simulink model "sim_6dof"  (R2025b)
settings: Solver=FixedStepAuto  StartTime=0.0  StopTime=30  FixedStep=0.005  RelTol=1e-3
InitFcn:
  | params_3dof
libraries: simulink_extras x1, simulink x1
settings Model: Creator=schwmaxi  LastModifiedBy=schwmaxi
settings OptimizationCC: UseDivisionForNetSlopeComputation=on  GainParamInheritBuiltInType=on  UseFloatMulNetSlope=on  EnhancedBackFolding=on  BooleansAsBitfields=on  PassReuseOutputArgsAs=Individual arguments  StateBitsets=on  DataBitsets=on  ZeroExternalMemoryAtStartup=off  ZeroInternalMemoryAtStartup=off  NoFixptDivByZeroProtection=on  EfficientFloat2IntCast=on  LifeSpan=1  OptimizeBlockOrder=speed  DifferentSizesBufferReuse=on  EfficientTunableParamExpr=on
settings DebuggingCC: ParameterTunabilityLossMsg=error
settings HardwareCC: ProdBitPerPointer=32.0  ProdBitPerSizeT=32.0  ProdBitPerPtrDiffT=32.0  ProdLargestAtomicFloat=None  ProdWordSize=32.0  ProdLongLongMode=on  ProdHWDeviceType=Custom Processor->Custom Processor
settings SFSimCC: MATLABDynamicMemAlloc=off  SimTargetLang=C++  SimDLTargetLibrary=mkl-dnn
settings RTWCC: SystemTargetFile=ert.tlc  GenCodeOnly=on  TemplateMakefile=ert_default_tmf  TargetLang=C++  Description=Embedded Coder
settings CodeAppCC: ForceParamTrailComments=on  IgnoreCustomStorageClasses=off  OperatorAnnotations=on  SimulinkDataObjDesc=on  SFDataObjDesc=on  CustomSymbolStrGlobalVar=rt$N$M  CustomSymbolStrType=$N$M  CustomSymbolStrFcn=$N$M$F  CustomSymbolStrMacro=$N$M  InsertBlockDesc=on
settings ERTTargetCC: InlinedParameterPlacement=Hierarchical  RootIOFormat=Structure reference  ERTCustomFileTemplate=example_file_process.tlc  ERTFilePackagingFormat=CompactWithDataFile  TargetLangStandard=C++11 (ISO)  GenerateSampleERTMain=on  IncludeMdlTerminateFcn=off  CombineSignalStateStructs=on  SupportAbsoluteTime=off  CodeInterfacePackaging=C++ class  SubcomponentCodeInterfacePackaging=C++ class  SupportComplex=off  SupportNonInlinedSFcns=on

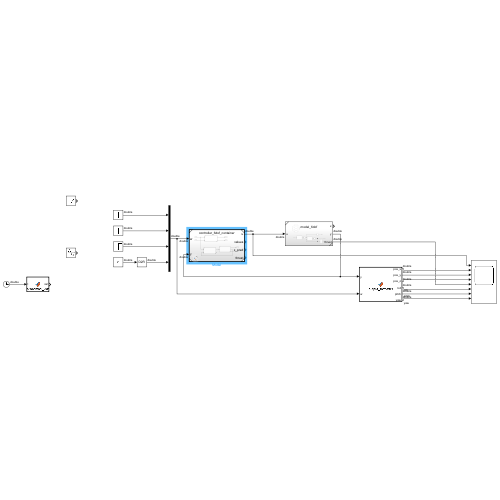
[thumbnail: Simulink's stored preview of the top-level diagram]
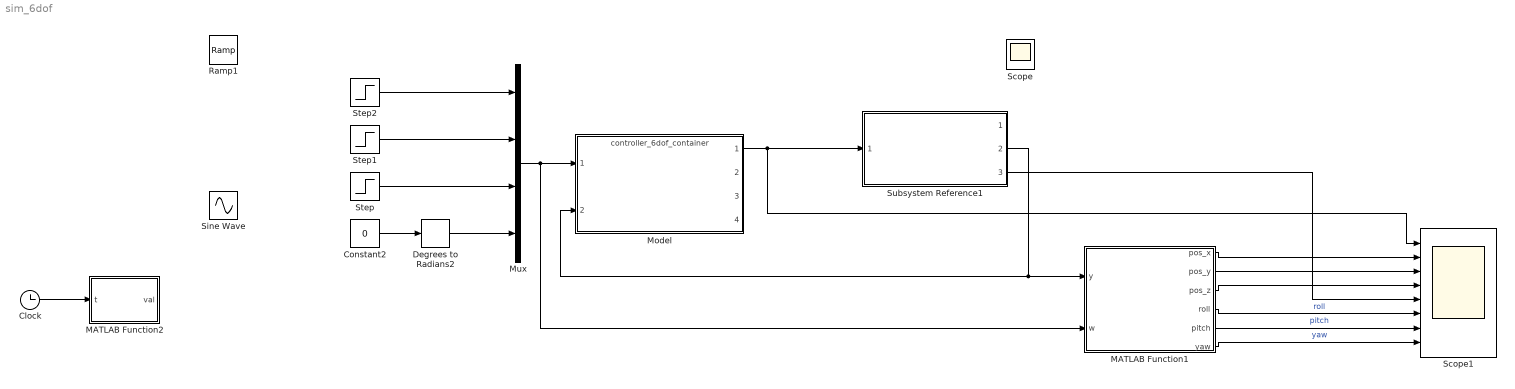
== system sim_6dof ==
  Clock : Clock
  Constant2 : Constant  Value=0
  Degrees to Radians2 : simulink_extras/Transformations/Degrees to Radians
  MATLAB Function1 : MATLAB Function  TreatAsAtomicUnit=on
  MATLAB Function2 : MATLAB Function  TreatAsAtomicUnit=on
  Model : ModelReference  ModelNameDialog=controller_6dof_container.slx  SimulationMode=Normal  ModelReferenceVersion=1.496
  Mux : Mux
  Ramp1 : simulink/Sources/Ramp  slope=-0.1  start=0  InitialOutput=0
  Scope1 : Scope  NumInputPorts=8
      settings: ActiveDisplayString=3  ActiveDisplayYMinimum=-0.079076952220866678  ActiveDisplayYMaximum=0.71169256998780028
  Sine Wave : Sin  Amplitude=5  Frequency=0.2 * 2 * pi  SampleTime=0
  Step : Step  After=0.05  SampleTime=0
  Step1 : Step  After=0.5  SampleTime=0
  Step2 : Step  After=0.5  SampleTime=0
  Subsystem Reference1 : Subsystem  ReferencedSubsystem=model_6dof
  Scope : Scope
      settings: ActiveDisplayYMinimum=-2.1631317412052181E+305  ActiveDisplayYMaximum=4.8211076094254489E+305  DataLoggingVariableName=ScopeData2
  wires:
  Constant2/1 -> Degrees to Radians2/1
  MATLAB Function1/4(roll) -> Scope1/6  "roll"
  MATLAB Function1/5(pitch) -> Scope1/7  "pitch"
  MATLAB Function1/6(yaw) -> Scope1/8  "yaw"
  Degrees to Radians2/1 -> Mux/4
  Clock/1 -> MATLAB Function2/1(t)
  Model/1 -> Scope1/1, Subsystem Reference1/1
  Mux/1 -> MATLAB Function1/2(w), Model/1
  Subsystem Reference1/2 -> MATLAB Function1/1(y), Model/2
  Step2/1 -> Mux/1
  Step1/1 -> Mux/2
  Step/1 -> Mux/3
  MATLAB Function1/1(pos_x) -> Scope1/2
  MATLAB Function1/2(pos_y) -> Scope1/3
  MATLAB Function1/3(pos_z) -> Scope1/4
  Subsystem Reference1/3 -> Scope1/5

== matlab function sim_6dof/MATLAB Function1 ==
  data: pos_x output; pos_y output; pos_z output; y input; w input; roll output; pitch output; yaw output
function [pos_x, pos_y, pos_z, roll, pitch, yaw] = output_formatter(y, w)
    pos_x = [w(1), y(1)];
    pos_y = [w(2), y(2)];
    pos_z = [w(3), y(3)];

    roll = y(4);
    pitch = y(5);
    yaw = y(6);
end

== matlab function sim_6dof/MATLAB Function2 ==
  data: t input; val output
function val = benchmark_30s(t)
    if t < 5
        val = 0.0;
    elseif t < 10
        val = 5.0;
    elseif t < 15
        val = 5.0 - 2 * (t - 10);
    elseif t < 25
        val = 5.0 * sin(0.2 * (t - 15)^2);
    elseif t <= 30
        val = 2.5 * cos(pi/5 * (t - 25)) + 2.5;
    else
        val = 0.0;
    end
end
